simulink model "six_rod_tensegrity_model_2021a"  (R2021a)
settings: Solver=ode45  StartTime=0  StopTime=Inf  RelTol=1e-1
values from neighbouring files (symbols this model uses):
  grivity_z = -9.80665    [code_for_6_rods_tensegrity.m]
  i = 19    [drive_params.m]
  Jsum = Jd + Jp + Jnagr    (= 9.27e-08)    [drive_params.m]
  km = 9.32 / 1000    (= 0.00932)    [drive_params.m]
  kpdr = 0.81    [drive_params.m]
  kw = 60 / (2*pi * 1020)    (= 0.00936205547599)    [drive_params.m]
  L = 0.14 / 1000    (= 0.00014)    [drive_params.m]
  load_mass = 0.5    [code_for_6_rods_tensegrity.m]
  plane_offset = -(rod_length/2 + 0.032 + rod_radius)    [code_for_6_rods_tensegrity.m]
  R = 5.3    [drive_params.m]
  rod_end_drive_offset = spool_active_length    (= 0.015)    [code_for_6_rods_tensegrity.m]
  rod_end_mass = 0.05    [code_for_6_rods_tensegrity.m]
  rod_end_mass_with_drive = 0.2    [code_for_6_rods_tensegrity.m]
  rod_mass = 0.028    [code_for_6_rods_tensegrity.m]
  rod_mass_with_drive = 0.038    [code_for_6_rods_tensegrity.m]
  rod_radius = 0.004    [code_for_6_rods_tensegrity.m]
undefined symbols (not defined in the file or in its folder): Left_end_cap_1_1, Left_end_cap_2_3, Left_end_cap_3_5, Left_end_cap_4_7, Left_end_cap_5_9, Left_end_cap_6_11, Right_end_cap_1_2, Right_end_cap_2_4, Right_end_cap_3_6, Right_end_cap_4_8, Right_end_cap_5_10, Right_end_cap_6_12, Rod_center_1, Rod_center_2, Rod_center_3, Rod_center_4, Rod_center_5, Rod_center_6, sigbuilder_block, X, Y, Z
libraries: sm_lib x403, nesl_utility x73
(part 3 of 5)

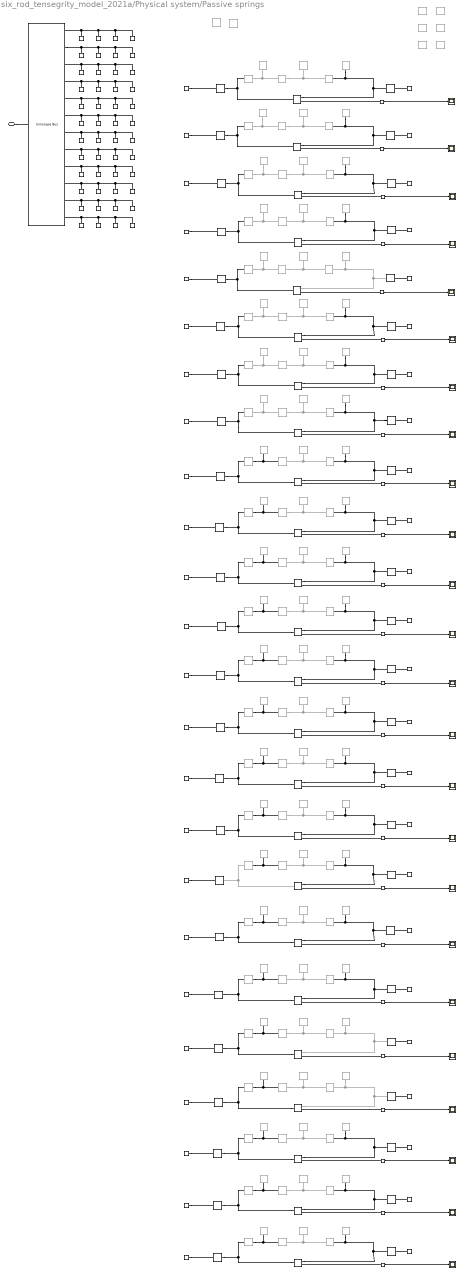
== system six_rod_tensegrity_model_2021a/Physical system/Passive springs ==
  note: Springs to passive rod
  note: Springs to active rod
  note: Springs to active rod
  note: Springs to passive rod
  note: Springs to passive rod
  note: Springs to active rod
  Cable properties {1..24} (24 alike) : sm_lib/Belts and Cables/Belt-Cable Properties  Commented=on  DrumBeltCableAlignment=Unrestricted  GraphicType=PitchLine  GraphicVisPropType=SimpleVisualProperties  GraphicDiffuseColor=cable_passive_color  GraphicSpecularColor=[0.5 0.5 0.5 1.0]  GraphicAmbientColor=[0.15 0.15 0.15 1.0]  GraphicEmissiveColor=[0.0 0.0 0.0 1.0]  GraphicShininess=75  GraphicOpacity=1
      settings: SourceProductBaseCode=MS
  Cable end {1..24} (24 alike) : sm_lib/Belts and Cables/Belt-Cable End  Commented=on
      settings: SourceProductBaseCode=MS
  Connection Label : ConnectionLabel  Label=Spring_left_1_1
  Connection Label1 : ConnectionLabel  Label=Spring_left_1_1
  Connection Label10 : ConnectionLabel  Label=Spring_left_7_2
  Connection Label11 : ConnectionLabel  Label=Spring_left_8_2
  Connection Label12 : ConnectionLabel  Label=Spring_left_7_2
  Connection Label13 : ConnectionLabel  Label=Spring_left_8_2
  Connection Label14 : ConnectionLabel  Label=Spring_left_5_2
  Connection Label15 : ConnectionLabel  Label=Spring_left_6_2
  Connection Label16 : ConnectionLabel  Label=Spring_left_9_3
  Connection Label17 : ConnectionLabel  Label=Spring_left_10_3
  Connection Label18 : ConnectionLabel  Label=Spring_left_11_3
  Connection Label19 : ConnectionLabel  Label=Spring_left_12_3
  Connection Label2 : ConnectionLabel  Label=Spring_left_2_1
  Connection Label20 : ConnectionLabel  Label=Spring_left_9_3
  Connection Label21 : ConnectionLabel  Label=Spring_left_10_3
  Connection Label22 : ConnectionLabel  Label=Spring_left_11_3
  Connection Label23 : ConnectionLabel  Label=Spring_left_12_3
  Connection Label24 : ConnectionLabel  Label=Spring_left_13_4
  Connection Label25 : ConnectionLabel  Label=Spring_left_14_4
  Connection Label26 : ConnectionLabel  Label=Spring_left_15_4
  Connection Label27 : ConnectionLabel  Label=Spring_left_16_4
  Connection Label28 : ConnectionLabel  Label=Spring_left_13_4
  Connection Label29 : ConnectionLabel  Label=Spring_left_14_4
  Connection Label3 : ConnectionLabel  Label=Spring_left_3_1
  Connection Label30 : ConnectionLabel  Label=Spring_left_15_4
  Connection Label31 : ConnectionLabel  Label=Spring_left_16_4
  Connection Label32 : ConnectionLabel  Label=Spring_left_17_5
  Connection Label33 : ConnectionLabel  Label=Spring_left_18_5
  Connection Label34 : ConnectionLabel  Label=Spring_left_19_6
  Connection Label35 : ConnectionLabel  Label=Spring_left_17_5
  Connection Label36 : ConnectionLabel  Label=Spring_left_18_5
  Connection Label37 : ConnectionLabel  Label=Spring_left_20_6
  Connection Label38 : ConnectionLabel  Label=Spring_left_19_6
  Connection Label39 : ConnectionLabel  Label=Spring_left_20_6
  Connection Label4 : ConnectionLabel  Label=Spring_left_4_1
  Connection Label40 : ConnectionLabel  Label=Spring_left_21_7
  Connection Label41 : ConnectionLabel  Label=Spring_left_22_7
  Connection Label42 : ConnectionLabel  Label=Spring_left_23_8
  Connection Label43 : ConnectionLabel  Label=Spring_left_24_8
  Connection Label44 : ConnectionLabel  Label=Spring_left_21_7
  Connection Label45 : ConnectionLabel  Label=Spring_left_22_7
  Connection Label46 : ConnectionLabel  Label=Spring_left_23_8
  Connection Label47 : ConnectionLabel  Label=Spring_left_24_8
  Connection Label48 : ConnectionLabel  Label=Spring_right_24_10
  Connection Label49 : ConnectionLabel  Label=Spring_right_23_9
  Connection Label5 : ConnectionLabel  Label=Spring_left_2_1
  Connection Label50 : ConnectionLabel  Label=Spring_right_22_12
  Connection Label51 : ConnectionLabel  Label=Spring_right_21_11
  Connection Label52 : ConnectionLabel  Label=Spring_right_20_10
  Connection Label53 : ConnectionLabel  Label=Spring_right_19_9
  Connection Label54 : ConnectionLabel  Label=Spring_right_18_12
  Connection Label55 : ConnectionLabel  Label=Spring_right_24_10
  Connection Label56 : ConnectionLabel  Label=Spring_right_23_9
  Connection Label57 : ConnectionLabel  Label=Spring_right_22_12
  Connection Label58 : ConnectionLabel  Label=Spring_right_21_11
  Connection Label59 : ConnectionLabel  Label=Spring_right_20_10
  Connection Label6 : ConnectionLabel  Label=Spring_left_3_1
  Connection Label60 : ConnectionLabel  Label=Spring_right_19_9
  Connection Label61 : ConnectionLabel  Label=Spring_right_18_12
  Connection Label62 : ConnectionLabel  Label=Spring_right_17_11
  Connection Label63 : ConnectionLabel  Label=Spring_right_16_12
  Connection Label64 : ConnectionLabel  Label=Spring_right_15_10
  Connection Label65 : ConnectionLabel  Label=Spring_right_14_8
  Connection Label66 : ConnectionLabel  Label=Spring_right_13_7
  Connection Label67 : ConnectionLabel  Label=Spring_right_12_12
  Connection Label68 : ConnectionLabel  Label=Spring_right_11_10
  Connection Label69 : ConnectionLabel  Label=Spring_right_10_6
  Connection Label7 : ConnectionLabel  Label=Spring_left_4_1
  Connection Label70 : ConnectionLabel  Label=Spring_right_9_5
  Connection Label71 : ConnectionLabel  Label=Spring_right_8_11
  Connection Label72 : ConnectionLabel  Label=Spring_right_7_9
  Connection Label73 : ConnectionLabel  Label=Spring_right_6_8
  Connection Label74 : ConnectionLabel  Label=Spring_right_5_7
  Connection Label75 : ConnectionLabel  Label=Spring_right_4_11
  Connection Label76 : ConnectionLabel  Label=Spring_right_3_9
  Connection Label77 : ConnectionLabel  Label=Spring_right_2_6
  Connection Label78 : ConnectionLabel  Label=Spring_right_1_5
  Connection Label79 : ConnectionLabel  Label=Spring_right_17_11
  Connection Label8 : ConnectionLabel  Label=Spring_left_5_2
  Connection Label80 : ConnectionLabel  Label=Spring_right_16_12
  Connection Label81 : ConnectionLabel  Label=Spring_right_15_10
  Connection Label82 : ConnectionLabel  Label=Spring_right_14_8
  Connection Label83 : ConnectionLabel  Label=Spring_right_13_7
  Connection Label84 : ConnectionLabel  Label=Spring_right_12_12
  Connection Label85 : ConnectionLabel  Label=Spring_right_11_10
  Connection Label86 : ConnectionLabel  Label=Spring_right_10_6
  Connection Label87 : ConnectionLabel  Label=Spring_right_9_5
  Connection Label88 : ConnectionLabel  Label=Spring_right_8_11
  Connection Label89 : ConnectionLabel  Label=Spring_right_7_9
  Connection Label9 : ConnectionLabel  Label=Spring_left_6_2
  Connection Label90 : ConnectionLabel  Label=Spring_right_6_8
  Connection Label91 : ConnectionLabel  Label=Spring_right_5_7
  Connection Label92 : ConnectionLabel  Label=Spring_right_4_11
  Connection Label93 : ConnectionLabel  Label=Spring_right_3_9
  Connection Label94 : ConnectionLabel  Label=Spring_right_2_6
  Connection Label95 : ConnectionLabel  Label=Spring_right_1_5
  End sphere {1..24} (24 alike) : sm_lib/Body Elements/Spherical Solid  Commented=on  GraphicAmbientColor=[0.15 0.15 0.15 1.0]  BasedOnType=Density  CenterOfMass=[0 0 0]  CenterOfMassUnits=m  GraphicDiffuseColor=spool_passive_color  Density=spool_passive_density  DensityUnits=kg/m^3  DoExposeReferenceFrame=on  GraphicEmissiveColor=[0.0 0.0 0.0 1.0]  ExportEntireGeometry=off  SerializedExposedGeometries=<ExposedGeometries/>  SerializedFrames=<Frames/>  MarkerShape=Frame  MarkerSize=10  GraphicType=FromGeometry  InertiaType=CalculateFromGeometry  Mass=0.01  MassUnits=kg  MomentsOfInertia=[1 1 1]  MomentsOfInertiaUnits=kg*m^2  GraphicOpacity=1.0  ProductsOfInertia=[0 0 0]  ProductsOfInertiaUnits=kg*m^2  GraphicShininess=10  GraphicSpecularColor=[0.8 0.8 0.8]  SphereRadius=spool_passive_radius  SphereRadiusUnits=m  GraphicVisPropType=SimpleVisualProperties
  PS-Simulink Converter{1..24} (24 alike) : nesl_utility/PS-Simulink Converter  PhysicalDomain=network_engine_domain  SubClassName=ps_output  LeftPortType=input  RightPortType=output  PseudoPeriodic=off  Frequencies=[]  Unit=N  AffineConversion=off
      settings: SourceProductBaseCode=PW,SS
  Revolute Joint {1..24} (24 alike) : sm_lib/Joints/Revolute Joint  Commented=on  JointMode=Normal  SenseConstraintForce=off  SenseConstraintForceX=off  SenseConstraintForceY=off  SenseConstraintForceZ=off  SenseConstraintTorque=off  SenseConstraintTorqueX=off  SenseConstraintTorqueY=off  SenseConstraintTorqueZ=off  SenseTotalForce=off  SenseTotalForceX=off  SenseTotalForceY=off  SenseTotalForceZ=off  SenseTotalTorque=off  SenseTotalTorqueX=off  SenseTotalTorqueY=off  SenseTotalTorqueZ=off  CompositeWrenchDir=FollowerOnBase  CompositeWrenchFrame=BaseFrame  EquilibriumPosition=0  EquilibriumPositionUnits=deg  SpringStiffness=0  SpringStiffnessUnits=N*m/deg  DampingCoefficient=0  DampingCoefficientUnits=N*m/(deg/s)  TorqueActuationMode=NoTorque  MotionActuationMode=ComputedMotion  SensePosition=off  SenseVelocity=off  SenseAcceleration=off  SenseTorqueForce=off  SenseLowerLimitTorqueForce=off  SenseUpperLimitTorqueForce=off  LowerLimitSpecify=off  LowerLimitBound=-90  LowerLimitBoundUnits=deg  LowerLimitStiffness=1e4  LowerLimitStiffnessUnits=N*m/deg  LowerLimitDamping=10  LowerLimitDampingUnits=N*m/(deg/s)  LowerLimitTransitionRegionWidth=0.1  LowerLimitTransitionRegionWidthUnits=deg  UpperLimitSpecify=off  UpperLimitBound=90  UpperLimitBoundUnits=deg  UpperLimitStiffness=1e4  UpperLimitStiffnessUnits=N*m/deg  UpperLimitDamping=10  UpperLimitDampingUnits=N*m/(deg/s)  UpperLimitTransitionRegionWidth=0.1  UpperLimitTransitionRegionWidthUnits=deg  PositionTargetSpecify=off  PositionTargetPriority=High  PositionTargetValue=0  PositionTargetValueUnits=deg  VelocityTargetSpecify=off  VelocityTargetPriority=High  VelocityTargetValue=0  VelocityTargetValueUnits=deg/s
  Simscape Bus1 : SimscapeBus  HierarchyStrings=Left_end_cap_1_1;Right_end_cap_1_2;Left_end_cap_2_3;Right_end_cap_2_4;Left_end_cap_3_5;Right_end_cap_3_6;Left_end_cap_4_7;Right_end_cap_4_8;Left_end_cap_5_9;Right_end_cap_5_10;Left_end_cap_6_11;Right_end_cap_6_12
  Sphere 1 : sm_lib/Body Elements/Spherical Solid  Commented=on  GraphicAmbientColor=[0.15 0.15 0.15 1.0]  BasedOnType=Density  CenterOfMass=[0 0 0]  CenterOfMassUnits=m  GraphicDiffuseColor=spool_passive_color  Density=spool_passive_density  DensityUnits=kg/m^3  DoExposeReferenceFrame=on  GraphicEmissiveColor=[0.0 0.0 0.0 1.0]  ExportEntireGeometry=off  SerializedExposedGeometries=<ExposedGeometries/>  SerializedFrames=<Frames/>  MarkerShape=Frame  MarkerSize=10  GraphicType=FromGeometry  InertiaType=CalculateFromGeometry  Mass=0.01  MassUnits=kg  MomentsOfInertia=[1 1 1]  MomentsOfInertiaUnits=kg*m^2  GraphicOpacity=1.0  ProductsOfInertia=[0 0 0]  ProductsOfInertiaUnits=kg*m^2  GraphicShininess=10  GraphicSpecularColor=[0.8 0.8 0.8]  SphereRadius=spool_passive_radius  SphereRadiusUnits=m  GraphicVisPropType=SimpleVisualProperties
  Spherical Joint 1 : sm_lib/Joints/Spherical Joint  Commented=on  JointMode=Normal  SenseConstraintForce=off  SenseConstraintForceX=off  SenseConstraintForceY=off  SenseConstraintForceZ=off  SenseConstraintTorque=off  SenseConstraintTorqueX=off  SenseConstraintTorqueY=off  SenseConstraintTorqueZ=off  SenseTotalForce=off  SenseTotalForceX=off  SenseTotalForceY=off  SenseTotalForceZ=off  SenseTotalTorque=off  SenseTotalTorqueX=off  SenseTotalTorqueY=off  SenseTotalTorqueZ=off  CompositeWrenchDir=FollowerOnBase  CompositeWrenchFrame=BaseFrame  DefPosRotationMethod=None  DefPosRotationAngleUnits=deg  DefPosRotationStandardAxis=+Z  DefPosRotationAngle=0.0  DefPosRotationArbitraryAxis=[0 0 1]  DefPosFollAlignAxisA=+X  DefPosBaseAlignAxisA=+Y  DefPosFollAlignAxisB=+Y  DefPosBaseAlignAxisB=+Z  DefPosRotationSequenceAxes=FollowerAxes  DefPosRotationSequence=XYX  DefPosRotationSequenceAngles=[0 0 0]  DefPosRotationSequenceAnglesUnits=deg  DefPosRotationMatrix=[1 0 0; 0 1 0; 0 0 1]  EqPosRotationMethod=None  EqPosRotationAngleUnits=deg  EqPosRotationStandardAxis=+Z  EqPosRotationAngle=0.0  EqPosRotationArbitraryAxis=[0 0 1]  EqPosFollAlignAxisA=+X  EqPosBaseAlignAxisA=+Y  EqPosFollAlignAxisB=+Y  EqPosBaseAlignAxisB=+Z  EqPosRotationSequenceAxes=FollowerAxes  EqPosRotationSequence=XYX  EqPosRotationSequenceAngles=[0 0 0]  EqPosRotationSequenceAnglesUnits=deg  EqPosRotationMatrix=[1 0 0; 0 1 0; 0 0 1]  SpringStiffness=0  SpringStiffnessUnits=N*m/deg  DampingCoefficient=0  DampingCoefficientUnits=N*m/(deg/s)  ActuateTorqueX=off  ActuateTorqueY=off  ActuateTorqueZ=off  ActuateTorque=off  TorqueActuationMode=NoTorque  MotionActuationMode=ComputedMotion  ActuationFrame=BaseFrame  SensePosition=off  SenseVelocityX=off  SenseVelocityY=off  SenseVelocityZ=off  SenseVelocity=off  SenseAccelerationX=off  SenseAccelerationY=off  SenseAccelerationZ=off  SenseAcceleration=off  SenseTorqueX=off  SenseTorqueY=off  SenseTorqueZ=off  SenseTorqueForce=off  SenseLowerLimitTorqueMag=off  SenseUpperLimitTorqueMag=off  SensingFrame=BaseFrame  LowerLimitSpecify=off  LowerLimitBound=15  LowerLimitBoundUnits=deg  LowerLimitStiffness=1e4  LowerLimitStiffnessUnits=N*m/deg  LowerLimitDamping=10  LowerLimitDampingUnits=N*m/(deg/s)  LowerLimitTransitionRegionWidth=0.1  LowerLimitTransitionRegionWidthUnits=deg  UpperLimitSpecify=off  UpperLimitBound=45  UpperLimitBoundUnits=deg  UpperLimitStiffness=1e4  UpperLimitStiffnessUnits=N*m/deg  UpperLimitDamping=10  UpperLimitDampingUnits=N*m/(deg/s)  UpperLimitTransitionRegionWidth=0.1  UpperLimitTransitionRegionWidthUnits=deg  PositionTargetRotationMethod=None  PositionTargetRotationAngleUnits=deg  PositionTargetRotationStandardAxis=+Z  PositionTargetRotationAngle=0.0  PositionTargetRotationArbitraryAxis=[0 0 1]  PositionTargetFollAlignAxisA=+X  PositionTargetBaseAlignAxisA=+Y  PositionTargetFollAlignAxisB=+Y  PositionTargetBaseAlignAxisB=+Z  PositionTargetRotationSequenceAxes=FollowerAxes  PositionTargetRotationSequence=XYX  PositionTargetRotationSequenceAngles=[0 0 0]  PositionTargetRotationSequenceAnglesUnits=deg  PositionTargetRotationMatrix=[1 0 0; 0 1 0; 0 0 1]  PositionTargetSpecify=off  PositionTargetPriority=High  VelocityTargetValue=[0 0 0]  VelocityTargetValueUnits=deg/s  VelocityTargetSpecify=off  VelocityTargetPriority=High  VelocityTargetInFollowerFrame=on
  Spool {1..24} (24 alike) : sm_lib/Belts and Cables/Belt-Cable Spool  Commented=on  PitchRadius=spool_passive_radius  PitchRadiusUnits=m  SenseSpoolAngleA=off  SenseFleetAngleA=off
      settings: SourceProductBaseCode=MS
  Spring 1 : sm_lib/Forces and Torques/Spring and Damper Force  NaturalLength=spring_natural_length_1  NaturalLengthUnits=m  SpringStiffness=spring_stiffness  SpringStiffnessUnits=N/m  DampingCoefficient=spring_damping  DampingCoefficientUnits=N/(m/s)  SenseForce=on
  Spring 10 : sm_lib/Forces and Torques/Spring and Damper Force  NaturalLength=spring_natural_length_10  NaturalLengthUnits=m  SpringStiffness=spring_stiffness  SpringStiffnessUnits=N/m  DampingCoefficient=spring_damping  DampingCoefficientUnits=N/(m/s)  SenseForce=on
  Spring 11 : sm_lib/Forces and Torques/Spring and Damper Force  NaturalLength=spring_natural_length_11  NaturalLengthUnits=m  SpringStiffness=spring_stiffness  SpringStiffnessUnits=N/m  DampingCoefficient=spring_damping  DampingCoefficientUnits=N/(m/s)  SenseForce=on
  Spring 12 : sm_lib/Forces and Torques/Spring and Damper Force  NaturalLength=spring_natural_length_12  NaturalLengthUnits=m  SpringStiffness=spring_stiffness  SpringStiffnessUnits=N/m  DampingCoefficient=spring_damping  DampingCoefficientUnits=N/(m/s)  SenseForce=on
  Spring 13 : sm_lib/Forces and Torques/Spring and Damper Force  NaturalLength=spring_natural_length_13  NaturalLengthUnits=m  SpringStiffness=spring_stiffness  SpringStiffnessUnits=N/m  DampingCoefficient=spring_damping  DampingCoefficientUnits=N/(m/s)  SenseForce=on
  Spring 14 : sm_lib/Forces and Torques/Spring and Damper Force  NaturalLength=spring_natural_length_14  NaturalLengthUnits=m  SpringStiffness=spring_stiffness  SpringStiffnessUnits=N/m  DampingCoefficient=spring_damping  DampingCoefficientUnits=N/(m/s)  SenseForce=on
  Spring 15 : sm_lib/Forces and Torques/Spring and Damper Force  NaturalLength=spring_natural_length_15  NaturalLengthUnits=m  SpringStiffness=spring_stiffness  SpringStiffnessUnits=N/m  DampingCoefficient=spring_damping  DampingCoefficientUnits=N/(m/s)  SenseForce=on
  Spring 16 : sm_lib/Forces and Torques/Spring and Damper Force  NaturalLength=spring_natural_length_16  NaturalLengthUnits=m  SpringStiffness=spring_stiffness  SpringStiffnessUnits=N/m  DampingCoefficient=spring_damping  DampingCoefficientUnits=N/(m/s)  SenseForce=on
  Spring 17 : sm_lib/Forces and Torques/Spring and Damper Force  NaturalLength=spring_natural_length_17  NaturalLengthUnits=m  SpringStiffness=spring_stiffness  SpringStiffnessUnits=N/m  DampingCoefficient=spring_damping  DampingCoefficientUnits=N/(m/s)  SenseForce=on
  Spring 18 : sm_lib/Forces and Torques/Spring and Damper Force  NaturalLength=spring_natural_length_18  NaturalLengthUnits=m  SpringStiffness=spring_stiffness  SpringStiffnessUnits=N/m  DampingCoefficient=spring_damping  DampingCoefficientUnits=N/(m/s)  SenseForce=on
  Spring 19 : sm_lib/Forces and Torques/Spring and Damper Force  NaturalLength=spring_natural_length_19  NaturalLengthUnits=m  SpringStiffness=spring_stiffness  SpringStiffnessUnits=N/m  DampingCoefficient=spring_damping  DampingCoefficientUnits=N/(m/s)  SenseForce=on
  Spring 2 : sm_lib/Forces and Torques/Spring and Damper Force  NaturalLength=spring_natural_length_2  NaturalLengthUnits=m  SpringStiffness=spring_stiffness  SpringStiffnessUnits=N/m  DampingCoefficient=spring_damping  DampingCoefficientUnits=N/(m/s)  SenseForce=on
  Spring 20 : sm_lib/Forces and Torques/Spring and Damper Force  NaturalLength=spring_natural_length_20  NaturalLengthUnits=m  SpringStiffness=spring_stiffness  SpringStiffnessUnits=N/m  DampingCoefficient=spring_damping  DampingCoefficientUnits=N/(m/s)  SenseForce=on
  Spring 21 : sm_lib/Forces and Torques/Spring and Damper Force  NaturalLength=spring_natural_length_21  NaturalLengthUnits=m  SpringStiffness=spring_stiffness  SpringStiffnessUnits=N/m  DampingCoefficient=spring_damping  DampingCoefficientUnits=N/(m/s)  SenseForce=on
  Spring 22 : sm_lib/Forces and Torques/Spring and Damper Force  NaturalLength=spring_natural_length_22  NaturalLengthUnits=m  SpringStiffness=spring_stiffness  SpringStiffnessUnits=N/m  DampingCoefficient=spring_damping  DampingCoefficientUnits=N/(m/s)  SenseForce=on
  Spring 23 : sm_lib/Forces and Torques/Spring and Damper Force  NaturalLength=spring_natural_length_23  NaturalLengthUnits=m  SpringStiffness=spring_stiffness  SpringStiffnessUnits=N/m  DampingCoefficient=spring_damping  DampingCoefficientUnits=N/(m/s)  SenseForce=on
  Spring 24 : sm_lib/Forces and Torques/Spring and Damper Force  NaturalLength=spring_natural_length_24  NaturalLengthUnits=m  SpringStiffness=spring_stiffness  SpringStiffnessUnits=N/m  DampingCoefficient=spring_damping  DampingCoefficientUnits=N/(m/s)  SenseForce=on
  Spring 3 : sm_lib/Forces and Torques/Spring and Damper Force  NaturalLength=spring_natural_length_3  NaturalLengthUnits=m  SpringStiffness=spring_stiffness  SpringStiffnessUnits=N/m  DampingCoefficient=spring_damping  DampingCoefficientUnits=N/(m/s)  SenseForce=on
  Spring 4 : sm_lib/Forces and Torques/Spring and Damper Force  NaturalLength=spring_natural_length_4  NaturalLengthUnits=m  SpringStiffness=spring_stiffness  SpringStiffnessUnits=N/m  DampingCoefficient=spring_damping  DampingCoefficientUnits=N/(m/s)  SenseForce=on
  Spring 5 : sm_lib/Forces and Torques/Spring and Damper Force  NaturalLength=spring_natural_length_5  NaturalLengthUnits=m  SpringStiffness=spring_stiffness  SpringStiffnessUnits=N/m  DampingCoefficient=spring_damping  DampingCoefficientUnits=N/(m/s)  SenseForce=on
  Spring 6 : sm_lib/Forces and Torques/Spring and Damper Force  NaturalLength=spring_natural_length_6  NaturalLengthUnits=m  SpringStiffness=spring_stiffness  SpringStiffnessUnits=N/m  DampingCoefficient=spring_damping  DampingCoefficientUnits=N/(m/s)  SenseForce=on
  Spring 7 : sm_lib/Forces and Torques/Spring and Damper Force  NaturalLength=spring_natural_length_7  NaturalLengthUnits=m  SpringStiffness=spring_stiffness  SpringStiffnessUnits=N/m  DampingCoefficient=spring_damping  DampingCoefficientUnits=N/(m/s)  SenseForce=on
  Spring 8 : sm_lib/Forces and Torques/Spring and Damper Force  NaturalLength=spring_natural_length_8  NaturalLengthUnits=m  SpringStiffness=spring_stiffness  SpringStiffnessUnits=N/m  DampingCoefficient=spring_damping  DampingCoefficientUnits=N/(m/s)  SenseForce=on
  Spring 9 : sm_lib/Forces and Torques/Spring and Damper Force  NaturalLength=spring_natural_length_9  NaturalLengthUnits=m  SpringStiffness=spring_stiffness  SpringStiffnessUnits=N/m  DampingCoefficient=spring_damping  DampingCoefficientUnits=N/(m/s)  SenseForce=on
  Winch {1..24} (24 alike) : sm_lib/Body Elements/Cylindrical Solid  Commented=on  GraphicAmbientColor=[0.15 0.15 0.15 1.0]  BasedOnType=Density  CenterOfMass=[0 0 0]  CenterOfMassUnits=m  GraphicDiffuseColor=spool_passive_color  CylinderLength=spool_passive_length  CylinderLengthUnits=m  CylinderRadius=spool_passive_radius  CylinderRadiusUnits=m  Density=spool_passive_density  DensityUnits=kg/m^3  DoExposeReferenceFrame=on  GraphicEmissiveColor=[0.0 0.0 0.0 1.0]  ExportEntireGeometry=off  SerializedFrames=<Frames/>  MarkerShape=Frame  MarkerSize=10  GraphicType=FromGeometry  InertiaType=CalculateFromGeometry  Mass=0.01  MassUnits=kg  MomentsOfInertia=[1 1 1]  MomentsOfInertiaUnits=kg*m^2  GraphicOpacity=1.0  ProductsOfInertia=[0 0 0]  ProductsOfInertiaUnits=kg*m^2  GraphicShininess=10  GraphicSpecularColor=[0.8 0.8 0.8]  GraphicVisPropType=SimpleVisualProperties
  X+1 : sm_lib/Frames and Transforms/Rigid Transform  TranslationMethod=StandardAxis  TranslationStandardOffset=rod_radius  TranslationLengthUnit=m  TranslationStandardAxis=+X  TranslationCartesianOffset=[0 0 0]  TranslationROffset=0  TranslationROffsetUnits=m  TranslationZOffset=0  TranslationZOffsetUnits=m  TranslationThetaOffset=0  TranslationThetaOffsetUnits=deg  RotationMethod=StandardAxis  RotationAngleUnits=deg  RotationStandardAxis=-X  RotationAngle=90  RotationArbitraryAxis=[0 0 1]  FollAlignAxisA=+X  BaseAlignAxisA=+Y  FollAlignAxisB=+Y  BaseAlignAxisB=+Z  RotationSequenceAxes=FollowerAxes  RotationSequence=XYX  RotationSequenceAngles=[0 0 0]  RotationSequenceAnglesUnits=deg  RotationMatrix=[1 0 0; 0 1 0; 0 0 1]
  X+{4..12} (9 alike) : sm_lib/Frames and Transforms/Rigid Transform  TranslationMethod=StandardAxis  TranslationStandardOffset=rod_radius  TranslationLengthUnit=m  TranslationStandardAxis=+X  TranslationCartesianOffset=[0 0 0]  TranslationROffset=0  TranslationROffsetUnits=m  TranslationZOffset=0  TranslationZOffsetUnits=m  TranslationThetaOffset=0  TranslationThetaOffsetUnits=deg  RotationMethod=None  RotationAngleUnits=deg  RotationStandardAxis=+Z  RotationAngle=0.0  RotationArbitraryAxis=[0 0 1]  FollAlignAxisA=+X  BaseAlignAxisA=+Y  FollAlignAxisB=+Y  BaseAlignAxisB=+Z  RotationSequenceAxes=FollowerAxes  RotationSequence=XYX  RotationSequenceAngles=[0 0 0]  RotationSequenceAnglesUnits=deg  RotationMatrix=[1 0 0; 0 1 0; 0 0 1]
  X+2 : sm_lib/Frames and Transforms/Rigid Transform  TranslationMethod=StandardAxis  TranslationStandardOffset=rod_radius  TranslationLengthUnit=m  TranslationStandardAxis=+X  TranslationCartesianOffset=[0 0 0]  TranslationROffset=0  TranslationROffsetUnits=m  TranslationZOffset=0  TranslationZOffsetUnits=m  TranslationThetaOffset=0  TranslationThetaOffsetUnits=deg  RotationMethod=StandardAxis  RotationAngleUnits=deg  RotationStandardAxis=+X  RotationAngle=90  RotationArbitraryAxis=[0 0 1]  FollAlignAxisA=+X  BaseAlignAxisA=+Y  FollAlignAxisB=+Y  BaseAlignAxisB=+Z  RotationSequenceAxes=FollowerAxes  RotationSequence=XYX  RotationSequenceAngles=[0 0 0]  RotationSequenceAnglesUnits=deg  RotationMatrix=[1 0 0; 0 1 0; 0 0 1]
  X+3 : sm_lib/Frames and Transforms/Rigid Transform  TranslationMethod=StandardAxis  TranslationStandardOffset=rod_radius  TranslationLengthUnit=m  TranslationStandardAxis=+X  TranslationCartesianOffset=[0 0 0]  TranslationROffset=0  TranslationROffsetUnits=m  TranslationZOffset=0  TranslationZOffsetUnits=m  TranslationThetaOffset=0  TranslationThetaOffsetUnits=deg  RotationMethod=StandardAxis  RotationAngleUnits=deg  RotationStandardAxis=-X  RotationAngle=90  RotationArbitraryAxis=[0 0 1]  FollAlignAxisA=+X  BaseAlignAxisA=+Y  FollAlignAxisB=+Y  BaseAlignAxisB=+Z  RotationSequenceAxes=FollowerAxes  RotationSequence=XYX  RotationSequenceAngles=[0 0 0]  RotationSequenceAnglesUnits=deg  RotationMatrix=[1 0 0; 0 1 0; 0 0 1]
  X+Temp : sm_lib/Frames and Transforms/Rigid Transform  Commented=on  TranslationMethod=StandardAxis  TranslationStandardOffset=rod_radius  TranslationLengthUnit=m  TranslationStandardAxis=+X  TranslationCartesianOffset=[0 0 0]  TranslationROffset=0  TranslationROffsetUnits=m  TranslationZOffset=0  TranslationZOffsetUnits=m  TranslationThetaOffset=0  TranslationThetaOffsetUnits=deg  RotationMethod=None  RotationAngleUnits=deg  RotationStandardAxis=+Z  RotationAngle=0.0  RotationArbitraryAxis=[0 0 1]  FollAlignAxisA=+X  BaseAlignAxisA=+Y  FollAlignAxisB=+Y  BaseAlignAxisB=+Z  RotationSequenceAxes=FollowerAxes  RotationSequence=XYX  RotationSequenceAngles=[0 0 0]  RotationSequenceAnglesUnits=deg  RotationMatrix=[1 0 0; 0 1 0; 0 0 1]
  X-1 : sm_lib/Frames and Transforms/Rigid Transform  TranslationMethod=StandardAxis  TranslationStandardOffset=rod_radius  TranslationLengthUnit=m  TranslationStandardAxis=-X  TranslationCartesianOffset=[0 0 0]  TranslationROffset=0  TranslationROffsetUnits=m  TranslationZOffset=0  TranslationZOffsetUnits=m  TranslationThetaOffset=0  TranslationThetaOffsetUnits=deg  RotationMethod=StandardAxis  RotationAngleUnits=deg  RotationStandardAxis=+X  RotationAngle=90  RotationArbitraryAxis=[0 0 1]  FollAlignAxisA=+X  BaseAlignAxisA=+Y  FollAlignAxisB=+Y  BaseAlignAxisB=+Z  RotationSequenceAxes=FollowerAxes  RotationSequence=XYX  RotationSequenceAngles=[0 0 0]  RotationSequenceAnglesUnits=deg  RotationMatrix=[1 0 0; 0 1 0; 0 0 1]
  X-{4..12} (9 alike) : sm_lib/Frames and Transforms/Rigid Transform  TranslationMethod=StandardAxis  TranslationStandardOffset=rod_radius  TranslationLengthUnit=m  TranslationStandardAxis=-X  TranslationCartesianOffset=[0 0 0]  TranslationROffset=0  TranslationROffsetUnits=m  TranslationZOffset=0  TranslationZOffsetUnits=m  TranslationThetaOffset=0  TranslationThetaOffsetUnits=deg  RotationMethod=None  RotationAngleUnits=deg  RotationStandardAxis=+Z  RotationAngle=0.0  RotationArbitraryAxis=[0 0 1]  FollAlignAxisA=+X  BaseAlignAxisA=+Y  FollAlignAxisB=+Y  BaseAlignAxisB=+Z  RotationSequenceAxes=FollowerAxes  RotationSequence=XYX  RotationSequenceAngles=[0 0 0]  RotationSequenceAnglesUnits=deg  RotationMatrix=[1 0 0; 0 1 0; 0 0 1]
  X-2 : sm_lib/Frames and Transforms/Rigid Transform  TranslationMethod=StandardAxis  TranslationStandardOffset=rod_radius  TranslationLengthUnit=m  TranslationStandardAxis=-X  TranslationCartesianOffset=[0 0 0]  TranslationROffset=0  TranslationROffsetUnits=m  TranslationZOffset=0  TranslationZOffsetUnits=m  TranslationThetaOffset=0  TranslationThetaOffsetUnits=deg  RotationMethod=StandardAxis  RotationAngleUnits=deg  RotationStandardAxis=-X  RotationAngle=90  RotationArbitraryAxis=[0 0 1]  FollAlignAxisA=+X  BaseAlignAxisA=+Y  FollAlignAxisB=+Y  BaseAlignAxisB=+Z  RotationSequenceAxes=FollowerAxes  RotationSequence=XYX  RotationSequenceAngles=[0 0 0]  RotationSequenceAnglesUnits=deg  RotationMatrix=[1 0 0; 0 1 0; 0 0 1]
  X-3 : sm_lib/Frames and Transforms/Rigid Transform  TranslationMethod=StandardAxis  TranslationStandardOffset=rod_radius  TranslationLengthUnit=m  TranslationStandardAxis=-X  TranslationCartesianOffset=[0 0 0]  TranslationROffset=0  TranslationROffsetUnits=m  TranslationZOffset=0  TranslationZOffsetUnits=m  TranslationThetaOffset=0  TranslationThetaOffsetUnits=deg  RotationMethod=StandardAxis  RotationAngleUnits=deg  RotationStandardAxis=+X  RotationAngle=90  RotationArbitraryAxis=[0 0 1]  FollAlignAxisA=+X  BaseAlignAxisA=+Y  FollAlignAxisB=+Y  BaseAlignAxisB=+Z  RotationSequenceAxes=FollowerAxes  RotationSequence=XYX  RotationSequenceAngles=[0 0 0]  RotationSequenceAnglesUnits=deg  RotationMatrix=[1 0 0; 0 1 0; 0 0 1]
  X-Temp : sm_lib/Frames and Transforms/Rigid Transform  Commented=on  TranslationMethod=StandardAxis  TranslationStandardOffset=rod_radius  TranslationLengthUnit=m  TranslationStandardAxis=-X  TranslationCartesianOffset=[0 0 0]  TranslationROffset=0  TranslationROffsetUnits=m  TranslationZOffset=0  TranslationZOffsetUnits=m  TranslationThetaOffset=0  TranslationThetaOffsetUnits=deg  RotationMethod=None  RotationAngleUnits=deg  RotationStandardAxis=+Z  RotationAngle=0.0  RotationArbitraryAxis=[0 0 1]  FollAlignAxisA=+X  BaseAlignAxisA=+Y  FollAlignAxisB=+Y  BaseAlignAxisB=+Z  RotationSequenceAxes=FollowerAxes  RotationSequence=XYX  RotationSequenceAngles=[0 0 0]  RotationSequenceAnglesUnits=deg  RotationMatrix=[1 0 0; 0 1 0; 0 0 1]
  Y+1 : sm_lib/Frames and Transforms/Rigid Transform  TranslationMethod=StandardAxis  TranslationStandardOffset=rod_radius  TranslationLengthUnit=m  TranslationStandardAxis=+Y  TranslationCartesianOffset=[0 0 0]  TranslationROffset=0  TranslationROffsetUnits=m  TranslationZOffset=0  TranslationZOffsetUnits=m  TranslationThetaOffset=0  TranslationThetaOffsetUnits=deg  RotationMethod=StandardAxis  RotationAngleUnits=deg  RotationStandardAxis=-Y  RotationAngle=90  RotationArbitraryAxis=[0 0 1]  FollAlignAxisA=+X  BaseAlignAxisA=+Y  FollAlignAxisB=+Y  BaseAlignAxisB=+Z  RotationSequenceAxes=FollowerAxes  RotationSequence=XYX  RotationSequenceAngles=[0 0 0]  RotationSequenceAnglesUnits=deg  RotationMatrix=[1 0 0; 0 1 0; 0 0 1]
  Y+{4,6..12} (8 alike) : sm_lib/Frames and Transforms/Rigid Transform  TranslationMethod=StandardAxis  TranslationStandardOffset=rod_radius  TranslationLengthUnit=m  TranslationStandardAxis=+Y  TranslationCartesianOffset=[0 0 0]  TranslationROffset=0  TranslationROffsetUnits=m  TranslationZOffset=0  TranslationZOffsetUnits=m  TranslationThetaOffset=0  TranslationThetaOffsetUnits=deg  RotationMethod=None  RotationAngleUnits=deg  RotationStandardAxis=+Z  RotationAngle=0.0  RotationArbitraryAxis=[0 0 1]  FollAlignAxisA=+X  BaseAlignAxisA=+Y  FollAlignAxisB=+Y  BaseAlignAxisB=+Z  RotationSequenceAxes=FollowerAxes  RotationSequence=XYX  RotationSequenceAngles=[0 0 0]  RotationSequenceAnglesUnits=deg  RotationMatrix=[1 0 0; 0 1 0; 0 0 1]
  Y+2 : sm_lib/Frames and Transforms/Rigid Transform  TranslationMethod=StandardAxis  TranslationStandardOffset=rod_radius  TranslationLengthUnit=m  TranslationStandardAxis=+Y  TranslationCartesianOffset=[0 0 0]  TranslationROffset=0  TranslationROffsetUnits=m  TranslationZOffset=0  TranslationZOffsetUnits=m  TranslationThetaOffset=0  TranslationThetaOffsetUnits=deg  RotationMethod=StandardAxis  RotationAngleUnits=deg  RotationStandardAxis=+Y  RotationAngle=90  RotationArbitraryAxis=[0 0 1]  FollAlignAxisA=+X  BaseAlignAxisA=+Y  FollAlignAxisB=+Y  BaseAlignAxisB=+Z  RotationSequenceAxes=FollowerAxes  RotationSequence=XYX  RotationSequenceAngles=[0 0 0]  RotationSequenceAnglesUnits=deg  RotationMatrix=[1 0 0; 0 1 0; 0 0 1]
  Y+3 : sm_lib/Frames and Transforms/Rigid Transform  TranslationMethod=StandardAxis  TranslationStandardOffset=rod_radius  TranslationLengthUnit=m  TranslationStandardAxis=+Y  TranslationCartesianOffset=[0 0 0]  TranslationROffset=0  TranslationROffsetUnits=m  TranslationZOffset=0  TranslationZOffsetUnits=m  TranslationThetaOffset=0  TranslationThetaOffsetUnits=deg  RotationMethod=StandardAxis  RotationAngleUnits=deg  RotationStandardAxis=-Y  RotationAngle=90  RotationArbitraryAxis=[0 0 1]  FollAlignAxisA=+X  BaseAlignAxisA=+Y  FollAlignAxisB=+Y  BaseAlignAxisB=+Z  RotationSequenceAxes=FollowerAxes  RotationSequence=XYX  RotationSequenceAngles=[0 0 0]  RotationSequenceAnglesUnits=deg  RotationMatrix=[1 0 0; 0 1 0; 0 0 1]
  Y+5 : sm_lib/Frames and Transforms/Rigid Transform  TranslationMethod=StandardAxis  TranslationStandardOffset=rod_radius  TranslationLengthUnit=m  TranslationStandardAxis=+Y  TranslationCartesianOffset=[0 0 0]  TranslationROffset=0  TranslationROffsetUnits=m  TranslationZOffset=0  TranslationZOffsetUnits=m  TranslationThetaOffset=0  TranslationThetaOffsetUnits=deg  RotationMethod=StandardAxis  RotationAngleUnits=deg  RotationStandardAxis=-Y  RotationAngle=90  RotationArbitraryAxis=[0 0 1]  FollAlignAxisA=+X  BaseAlignAxisA=+Y  FollAlignAxisB=+Y  BaseAlignAxisB=+Z  RotationSequenceAxes=FollowerAxes  RotationSequence=XYX  RotationSequenceAngles=[0 0 0]  RotationSequenceAnglesUnits=deg  RotationMatrix=[1 0 0; 0 1 0; 0 0 1]
  Y+Temp : sm_lib/Frames and Transforms/Rigid Transform  Commented=on  TranslationMethod=StandardAxis  TranslationStandardOffset=rod_radius  TranslationLengthUnit=m  TranslationStandardAxis=+Y  TranslationCartesianOffset=[0 0 0]  TranslationROffset=0  TranslationROffsetUnits=m  TranslationZOffset=0  TranslationZOffsetUnits=m  TranslationThetaOffset=0  TranslationThetaOffsetUnits=deg  RotationMethod=None  RotationAngleUnits=deg  RotationStandardAxis=+Z  RotationAngle=0.0  RotationArbitraryAxis=[0 0 1]  FollAlignAxisA=+X  BaseAlignAxisA=+Y  FollAlignAxisB=+Y  BaseAlignAxisB=+Z  RotationSequenceAxes=FollowerAxes  RotationSequence=XYX  RotationSequenceAngles=[0 0 0]  RotationSequenceAnglesUnits=deg  RotationMatrix=[1 0 0; 0 1 0; 0 0 1]
  Y-1 : sm_lib/Frames and Transforms/Rigid Transform  TranslationMethod=StandardAxis  TranslationStandardOffset=rod_radius  TranslationLengthUnit=m  TranslationStandardAxis=-Y  TranslationCartesianOffset=[0 0 0]  TranslationROffset=0  TranslationROffsetUnits=m  TranslationZOffset=0  TranslationZOffsetUnits=m  TranslationThetaOffset=0  TranslationThetaOffsetUnits=deg  RotationMethod=StandardAxis  RotationAngleUnits=deg  RotationStandardAxis=+Y  RotationAngle=90  RotationArbitraryAxis=[0 0 1]  FollAlignAxisA=+X  BaseAlignAxisA=+Y  FollAlignAxisB=+Y  BaseAlignAxisB=+Z  RotationSequenceAxes=FollowerAxes  RotationSequence=XYX  RotationSequenceAngles=[0 0 0]  RotationSequenceAnglesUnits=deg  RotationMatrix=[1 0 0; 0 1 0; 0 0 1]
  Y-{4,6..12} (8 alike) : sm_lib/Frames and Transforms/Rigid Transform  TranslationMethod=StandardAxis  TranslationStandardOffset=rod_radius  TranslationLengthUnit=m  TranslationStandardAxis=-Y  TranslationCartesianOffset=[0 0 0]  TranslationROffset=0  TranslationROffsetUnits=m  TranslationZOffset=0  TranslationZOffsetUnits=m  TranslationThetaOffset=0  TranslationThetaOffsetUnits=deg  RotationMethod=None  RotationAngleUnits=deg  RotationStandardAxis=+Z  RotationAngle=0.0  RotationArbitraryAxis=[0 0 1]  FollAlignAxisA=+X  BaseAlignAxisA=+Y  FollAlignAxisB=+Y  BaseAlignAxisB=+Z  RotationSequenceAxes=FollowerAxes  RotationSequence=XYX  RotationSequenceAngles=[0 0 0]  RotationSequenceAnglesUnits=deg  RotationMatrix=[1 0 0; 0 1 0; 0 0 1]
  Y-2 : sm_lib/Frames and Transforms/Rigid Transform  TranslationMethod=StandardAxis  TranslationStandardOffset=rod_radius  TranslationLengthUnit=m  TranslationStandardAxis=-Y  TranslationCartesianOffset=[0 0 0]  TranslationROffset=0  TranslationROffsetUnits=m  TranslationZOffset=0  TranslationZOffsetUnits=m  TranslationThetaOffset=0  TranslationThetaOffsetUnits=deg  RotationMethod=StandardAxis  RotationAngleUnits=deg  RotationStandardAxis=-Y  RotationAngle=90  RotationArbitraryAxis=[0 0 1]  FollAlignAxisA=+X  BaseAlignAxisA=+Y  FollAlignAxisB=+Y  BaseAlignAxisB=+Z  RotationSequenceAxes=FollowerAxes  RotationSequence=XYX  RotationSequenceAngles=[0 0 0]  RotationSequenceAnglesUnits=deg  RotationMatrix=[1 0 0; 0 1 0; 0 0 1]
  Y-3 : sm_lib/Frames and Transforms/Rigid Transform  TranslationMethod=StandardAxis  TranslationStandardOffset=rod_radius  TranslationLengthUnit=m  TranslationStandardAxis=-Y  TranslationCartesianOffset=[0 0 0]  TranslationROffset=0  TranslationROffsetUnits=m  TranslationZOffset=0  TranslationZOffsetUnits=m  TranslationThetaOffset=0  TranslationThetaOffsetUnits=deg  RotationMethod=StandardAxis  RotationAngleUnits=deg  RotationStandardAxis=+Y  RotationAngle=90  RotationArbitraryAxis=[0 0 1]  FollAlignAxisA=+X  BaseAlignAxisA=+Y  FollAlignAxisB=+Y  BaseAlignAxisB=+Z  RotationSequenceAxes=FollowerAxes  RotationSequence=XYX  RotationSequenceAngles=[0 0 0]  RotationSequenceAnglesUnits=deg  RotationMatrix=[1 0 0; 0 1 0; 0 0 1]
  Y-5 : sm_lib/Frames and Transforms/Rigid Transform  TranslationMethod=StandardAxis  TranslationStandardOffset=rod_radius  TranslationLengthUnit=m  TranslationStandardAxis=-Y  TranslationCartesianOffset=[0 0 0]  TranslationROffset=0  TranslationROffsetUnits=m  TranslationZOffset=0  TranslationZOffsetUnits=m  TranslationThetaOffset=0  TranslationThetaOffsetUnits=deg  RotationMethod=StandardAxis  RotationAngleUnits=deg  RotationStandardAxis=-Y  RotationAngle=90  RotationArbitraryAxis=[0 0 1]  FollAlignAxisA=+X  BaseAlignAxisA=+Y  FollAlignAxisB=+Y  BaseAlignAxisB=+Z  RotationSequenceAxes=FollowerAxes  RotationSequence=XYX  RotationSequenceAngles=[0 0 0]  RotationSequenceAnglesUnits=deg  RotationMatrix=[1 0 0; 0 1 0; 0 0 1]
  Y-Temp : sm_lib/Frames and Transforms/Rigid Transform  Commented=on  TranslationMethod=StandardAxis  TranslationStandardOffset=rod_radius  TranslationLengthUnit=m  TranslationStandardAxis=-Y  TranslationCartesianOffset=[0 0 0]  TranslationROffset=0  TranslationROffsetUnits=m  TranslationZOffset=0  TranslationZOffsetUnits=m  TranslationThetaOffset=0  TranslationThetaOffsetUnits=deg  RotationMethod=None  RotationAngleUnits=deg  RotationStandardAxis=+Z  RotationAngle=0.0  RotationArbitraryAxis=[0 0 1]  FollAlignAxisA=+X  BaseAlignAxisA=+Y  FollAlignAxisB=+Y  BaseAlignAxisB=+Z  RotationSequenceAxes=FollowerAxes  RotationSequence=XYX  RotationSequenceAngles=[0 0 0]  RotationSequenceAnglesUnits=deg  RotationMatrix=[1 0 0; 0 1 0; 0 0 1]
  Z+Temp : sm_lib/Frames and Transforms/Rigid Transform  Commented=on  TranslationMethod=StandardAxis  TranslationStandardOffset=rod_radius  TranslationLengthUnit=m  TranslationStandardAxis=+Z  TranslationCartesianOffset=[0 0 0]  TranslationROffset=0  TranslationROffsetUnits=m  TranslationZOffset=0  TranslationZOffsetUnits=m  TranslationThetaOffset=0  TranslationThetaOffsetUnits=deg  RotationMethod=None  RotationAngleUnits=deg  RotationStandardAxis=+Z  RotationAngle=0.0  RotationArbitraryAxis=[0 0 1]  FollAlignAxisA=+X  BaseAlignAxisA=+Y  FollAlignAxisB=+Y  BaseAlignAxisB=+Z  RotationSequenceAxes=FollowerAxes  RotationSequence=XYX  RotationSequenceAngles=[0 0 0]  RotationSequenceAnglesUnits=deg  RotationMatrix=[1 0 0; 0 1 0; 0 0 1]
  Z-Temp : sm_lib/Frames and Transforms/Rigid Transform  Commented=on  TranslationMethod=StandardAxis  TranslationStandardOffset=rod_radius  TranslationLengthUnit=m  TranslationStandardAxis=-Z  TranslationCartesianOffset=[0 0 0]  TranslationROffset=0  TranslationROffsetUnits=m  TranslationZOffset=0  TranslationZOffsetUnits=m  TranslationThetaOffset=0  TranslationThetaOffsetUnits=deg  RotationMethod=None  RotationAngleUnits=deg  RotationStandardAxis=+Z  RotationAngle=0.0  RotationArbitraryAxis=[0 0 1]  FollAlignAxisA=+X  BaseAlignAxisA=+Y  FollAlignAxisB=+Y  BaseAlignAxisB=+Z  RotationSequenceAxes=FollowerAxes  RotationSequence=XYX  RotationSequenceAngles=[0 0 0]  RotationSequenceAnglesUnits=deg  RotationMatrix=[1 0 0; 0 1 0; 0 0 1]
  spring force {1..24} (24 alike) : Scope
  Rods end caps bus : PMIOPort  Side=Left
  wires:
  PS-Simulink Converter1/1 -> spring force 1/1
  PS-Simulink Converter2/1 -> spring force 2/1
  PS-Simulink Converter3/1 -> spring force 3/1
  PS-Simulink Converter4/1 -> spring force 4/1
  PS-Simulink Converter5/1 -> spring force 5/1
  PS-Simulink Converter6/1 -> spring force 6/1
  PS-Simulink Converter7/1 -> spring force 7/1
  PS-Simulink Converter8/1 -> spring force 8/1
  PS-Simulink Converter9/1 -> spring force 9/1
  PS-Simulink Converter10/1 -> spring force 10/1
  PS-Simulink Converter11/1 -> spring force 11/1
  PS-Simulink Converter12/1 -> spring force 12/1
  PS-Simulink Converter13/1 -> spring force 13/1
  PS-Simulink Converter14/1 -> spring force 14/1
  PS-Simulink Converter15/1 -> spring force 15/1
  PS-Simulink Converter16/1 -> spring force 16/1
  PS-Simulink Converter17/1 -> spring force 17/1
  PS-Simulink Converter18/1 -> spring force 18/1
  PS-Simulink Converter19/1 -> spring force 19/1
  PS-Simulink Converter20/1 -> spring force 20/1
  PS-Simulink Converter21/1 -> spring force 21/1
  PS-Simulink Converter22/1 -> spring force 22/1
  PS-Simulink Converter23/1 -> spring force 23/1
  PS-Simulink Converter24/1 -> spring force 24/1
  connections:
  Connection Label/LConn1 -- Y+1/LConn1
  Connection Label3/LConn1 -- Y-1/LConn1
  Connection Label4/LConn1 -- X-1/LConn1
  Connection Label8/LConn1 -- Y+2/LConn1
  Connection Label10/LConn1 -- Y-2/LConn1
  Connection Label11/LConn1 -- X-2/LConn1
  Connection Label2/LConn1 -- X+1/LConn1
  Connection Label9/LConn1 -- X+2/LConn1
  Y+1/RConn1 -- Revolute Joint 1/LConn1 -- Spring 1/LConn1
  Spool 1/RConn1 -- Cable end 1/RConn1 -- Cable properties 1/LConn1
  Spool 1/LConn1 -- Revolute Joint 1/RConn1 -- Winch 1/RConn1
  Spring 1/RConn1 -- Y-5/RConn1 -- End sphere 1/RConn1 -- Cable end 1/LConn1
  PS-Simulink Converter1/LConn1 -- Spring 1/RConn2
  X+1/RConn1 -- Revolute Joint 2/LConn1 -- Spring 2/LConn1
  Y-6/RConn1 -- Spring 2/RConn1 -- End sphere 2/RConn1 -- Cable end 2/LConn1
  Spool 2/RConn1 -- Cable end 2/RConn1 -- Cable properties 2/LConn1
  Spool 2/LConn1 -- Revolute Joint 2/RConn1 -- Winch 2/RConn1
  PS-Simulink Converter2/LConn1 -- Spring 2/RConn2
  Y-1/RConn1 -- Revolute Joint 3/LConn1 -- Spring 3/LConn1
  Connection Label76/LConn1 -- X+9/LConn1
  Spool 3/RConn1 -- Cable end 3/RConn1 -- Cable properties 3/LConn1
  Spool 3/LConn1 -- Winch 3/RConn1 -- Revolute Joint 3/RConn1
  PS-Simulink Converter3/LConn1 -- Spring 3/RConn2
  X-1/RConn1 -- Revolute Joint 4/LConn1 -- Spring 4/LConn1
  Spring 4/RConn1 -- End sphere 4/RConn1 -- Cable end 4/LConn1 -- X-11/RConn1
  Spool 4/RConn1 -- Cable end 4/RConn1 -- Cable properties 4/LConn1
  Spool 4/LConn1 -- Winch 4/RConn1 -- Revolute Joint 4/RConn1
  PS-Simulink Converter4/LConn1 -- Spring 4/RConn2
  Y+2/RConn1 -- Revolute Joint 5/LConn1 -- Spring 5/LConn1
  Connection Label74/LConn1 -- X-7/LConn1
  Spool 5/RConn1 -- Cable end 5/RConn1 -- Cable properties 5/LConn1
  Spool 5/LConn1 -- Winch 5/RConn1 -- Revolute Joint 5/RConn1
  PS-Simulink Converter5/LConn1 -- Spring 5/RConn2
  X+2/RConn1 -- Revolute Joint 6/LConn1 -- Spring 6/LConn1
  Connection Label73/LConn1 -- X-8/LConn1
  Spool 6/RConn1 -- Cable end 6/RConn1 -- Cable properties 6/LConn1
  Spool 6/LConn1 -- Revolute Joint 6/RConn1 -- Winch 6/RConn1
  PS-Simulink Converter6/LConn1 -- Spring 6/RConn2
  Y-2/RConn1 -- Revolute Joint 7/LConn1 -- Spring 7/LConn1
  Y+9/RConn1 -- Spring 7/RConn1 -- End sphere 7/RConn1 -- Cable end 7/LConn1
  Spool 7/RConn1 -- Cable end 7/RConn1 -- Cable properties 7/LConn1
  Spool 7/LConn1 -- Winch 7/RConn1 -- Revolute Joint 7/RConn1
  PS-Simulink Converter7/LConn1 -- Spring 7/RConn2
  X-2/RConn1 -- Revolute Joint 8/LConn1 -- Spring 8/LConn1
  Connection Label71/LConn1 -- Y+11/LConn1
  Spool 8/RConn1 -- Cable end 8/RConn1 -- Cable properties 8/LConn1
  Spool 8/LConn1 -- Winch 8/RConn1 -- Revolute Joint 8/RConn1
  PS-Simulink Converter8/LConn1 -- Spring 8/RConn2
  Spring 9/LConn1 -- Y+3/RConn1 -- Revolute Joint 9/LConn1
  Connection Label70/LConn1 -- Y+5/LConn1
  Spool 9/RConn1 -- Cable end 9/RConn1 -- Cable properties 9/LConn1
  Winch 9/RConn1 -- Revolute Joint 9/RConn1 -- Spool 9/LConn1
  PS-Simulink Converter9/LConn1 -- Spring 9/RConn2
  Spring 10/LConn1 -- X-3/RConn1 -- Revolute Joint 10/LConn1
  Spring 10/RConn1 -- X+6/RConn1 -- End sphere 10/RConn1 -- Cable end 10/LConn1
  Spool 10/RConn1 -- Cable end 10/RConn1 -- Cable properties 10/LConn1
  Winch 10/RConn1 -- Revolute Joint 10/RConn1 -- Spool 10/LConn1
  PS-Simulink Converter10/LConn1 -- Spring 10/RConn2
  Spring 11/LConn1 -- Y-3/RConn1 -- Revolute Joint 11/LConn1
  Y-10/RConn1 -- Spring 11/RConn1 -- End sphere 11/RConn1 -- Cable end 11/LConn1
  Spool 11/RConn1 -- Cable end 11/RConn1 -- Cable properties 11/LConn1
  Winch 11/RConn1 -- Revolute Joint 11/RConn1 -- Spool 11/LConn1
  PS-Simulink Converter11/LConn1 -- Spring 11/RConn2
  Spring 12/LConn1 -- X+3/RConn1 -- Revolute Joint 12/LConn1
  Y-12/RConn1 -- Spring 12/RConn1 -- End sphere 12/RConn1 -- Cable end 12/LConn1
  Spool 12/RConn1 -- Cable end 12/RConn1 -- Cable properties 12/LConn1
  Winch 12/RConn1 -- Revolute Joint 12/RConn1 -- Spool 12/LConn1
  PS-Simulink Converter12/LConn1 -- Spring 12/RConn2
  Spring 13/LConn1 -- Y+4/RConn1 -- Revolute Joint 13/LConn1
  Y+7/RConn1 -- Spring 13/RConn1 -- End sphere 13/RConn1 -- Cable end 13/LConn1
  Spool 13/RConn1 -- Cable end 13/RConn1 -- Cable properties 13/LConn1
  Winch 13/RConn1 -- Revolute Joint 13/RConn1 -- Spool 13/LConn1
  PS-Simulink Converter13/LConn1 -- Spring 13/RConn2
  Spring 14/LConn1 -- X-4/RConn1 -- Revolute Joint 14/LConn1
  Y+8/RConn1 -- Spring 14/RConn1 -- End sphere 14/RConn1 -- Cable end 14/LConn1
  Spool 14/RConn1 -- Cable end 14/RConn1 -- Cable properties 14/LConn1
  Winch 14/RConn1 -- Revolute Joint 14/RConn1 -- Spool 14/LConn1
  PS-Simulink Converter14/LConn1 -- Spring 14/RConn2
  Spring 15/LConn1 -- Y-4/RConn1 -- Revolute Joint 15/LConn1
  X+10/RConn1 -- Spring 15/RConn1 -- End sphere 15/RConn1 -- Cable end 15/LConn1
  Spool 15/RConn1 -- Cable end 15/RConn1 -- Cable properties 15/LConn1
  Winch 15/RConn1 -- Revolute Joint 15/RConn1 -- Spool 15/LConn1
  PS-Simulink Converter15/LConn1 -- Spring 15/RConn2
  Connection Label27/LConn1 -- X+4/LConn1
  X-12/RConn1 -- Spring 16/RConn1 -- End sphere 16/RConn1 -- Cable end 16/LConn1
  Spool 16/RConn1 -- Cable end 16/RConn1 -- Cable properties 16/LConn1
  Winch 16/RConn1 -- Revolute Joint 16/RConn1 -- Spool 16/LConn1
  PS-Simulink Converter16/LConn1 -- Spring 16/RConn2
  Connection Label62/LConn1 -- Y-11/LConn1
  Spool 17/RConn1 -- Cable end 17/RConn1 -- Cable properties 17/LConn1
  Winch 17/RConn1 -- Revolute Joint 17/RConn1 -- Spool 17/LConn1
  PS-Simulink Converter17/LConn1 -- Spring 17/RConn2
  Spring 18/LConn1 -- X+5/RConn1 -- Revolute Joint 18/LConn1
  Connection Label54/LConn1 -- X+12/LConn1
  Spool 18/RConn1 -- Cable end 18/RConn1 -- Cable properties 18/LConn1
  Winch 18/RConn1 -- Revolute Joint 18/RConn1 -- Spool 18/LConn1
  PS-Simulink Converter18/LConn1 -- Spring 18/RConn2
  Spring 19/LConn1 -- X-6/RConn1 -- Revolute Joint 19/LConn1
  Y-9/RConn1 -- Spring 19/RConn1 -- End sphere 19/RConn1 -- Cable end 19/LConn1
  Spool 19/RConn1 -- Cable end 19/RConn1 -- Cable properties 19/LConn1
  Winch 19/RConn1 -- Revolute Joint 19/RConn1 -- Spool 19/LConn1
  PS-Simulink Converter19/LConn1 -- Spring 19/RConn2
  Spring 20/LConn1 -- Y+6/RConn1 -- Revolute Joint 20/LConn1
  Connection Label52/LConn1 -- X-10/LConn1
  Spool 20/RConn1 -- Cable end 20/RConn1 -- Cable properties 20/LConn1
  Winch 20/RConn1 -- Revolute Joint 20/RConn1 -- Spool 20/LConn1
  PS-Simulink Converter20/LConn1 -- Spring 20/RConn2
  Spring 21/LConn1 -- Y-7/RConn1 -- Revolute Joint 21/LConn1
  Connection Label51/LConn1 -- X+11/LConn1
  Spool 21/RConn1 -- Cable end 21/RConn1 -- Cable properties 21/LConn1
  Winch 21/RConn1 -- Revolute Joint 21/RConn1 -- Spool 21/LConn1
  PS-Simulink Converter21/LConn1 -- Spring 21/RConn2
  Spring 22/LConn1 -- X+7/RConn1 -- Revolute Joint 22/LConn1
  Y+12/RConn1 -- Spring 22/RConn1 -- End sphere 22/RConn1 -- Cable end 22/LConn1
  Spool 22/RConn1 -- Cable end 22/RConn1 -- Cable properties 22/LConn1
  Winch 22/RConn1 -- Revolute Joint 22/RConn1 -- Spool 22/LConn1
  PS-Simulink Converter22/LConn1 -- Spring 22/RConn2
  Spring 23/LConn1 -- Y-8/RConn1 -- Revolute Joint 23/LConn1
  X-9/RConn1 -- Spring 23/RConn1 -- End sphere 23/RConn1 -- Cable end 23/LConn1
  Spool 23/RConn1 -- Cable end 23/RConn1 -- Cable properties 23/LConn1
  Winch 23/RConn1 -- Revolute Joint 23/RConn1 -- Spool 23/LConn1
  PS-Simulink Converter23/LConn1 -- Spring 23/RConn2
  Spring 24/LConn1 -- X+8/RConn1 -- Revolute Joint 24/LConn1
  Connection Label48/LConn1 -- Y+10/LConn1
  Spool 24/RConn1 -- Cable end 24/RConn1 -- Cable properties 24/LConn1
  Winch 24/RConn1 -- Revolute Joint 24/RConn1 -- Spool 24/LConn1
  PS-Simulink Converter24/LConn1 -- Spring 24/RConn2
  Connection Label19/LConn1 -- X+3/LConn1
  Connection Label18/LConn1 -- Y-3/LConn1
  Connection Label17/LConn1 -- X-3/LConn1
  Connection Label16/LConn1 -- Y+3/LConn1
  X+4/RConn1 -- Revolute Joint 16/LConn1 -- Spring 16/LConn1
  Connection Label25/LConn1 -- X-4/LConn1
  Connection Label26/LConn1 -- Y-4/LConn1
  Connection Label24/LConn1 -- Y+4/LConn1
  Spring 9/RConn1 -- Y+5/RConn1 -- End sphere 9/RConn1 -- Cable end 9/LConn1
  Connection Label78/LConn1 -- Y-5/LConn1
  Connection Label33/LConn1 -- X+5/LConn1
  Revolute Joint 17/LConn1 -- X-5/RConn1 -- Spring 17/LConn1
  Connection Label34/LConn1 -- X-6/LConn1
  Connection Label69/LConn1 -- X+6/LConn1
  Connection Label37/LConn1 -- Y+6/LConn1
  Connection Label77/LConn1 -- Y-6/LConn1
  Connection Label40/LConn1 -- Y-7/LConn1
  Connection Label66/LConn1 -- Y+7/LConn1
  End sphere 5/RConn1 -- Cable end 5/LConn1 -- Spring 5/RConn1 -- X-7/RConn1
  Connection Label41/LConn1 -- X+7/LConn1
  Connection Label43/LConn1 -- X+8/LConn1
  X-8/RConn1 -- Spring 6/RConn1 -- End sphere 6/RConn1 -- Cable end 6/LConn1
  Connection Label42/LConn1 -- Y-8/LConn1
  Connection Label65/LConn1 -- Y+8/LConn1
  X+9/RConn1 -- Spring 3/RConn1 -- End sphere 3/RConn1 -- Cable end 3/LConn1
  Connection Label49/LConn1 -- X-9/LConn1
  Connection Label72/LConn1 -- Y+9/LConn1
  Connection Label53/LConn1 -- Y-9/LConn1
  Connection Label64/LConn1 -- X+10/LConn1
  End sphere 20/RConn1 -- Cable end 20/LConn1 -- X-10/RConn1 -- Spring 20/RConn1
  Y+10/RConn1 -- Spring 24/RConn1 -- End sphere 24/RConn1 -- Cable end 24/LConn1
  Connection Label68/LConn1 -- Y-10/LConn1
  End sphere 21/RConn1 -- Cable end 21/LConn1 -- X+11/RConn1 -- Spring 21/RConn1
  Connection Label75/LConn1 -- X-11/LConn1
  Spring 8/RConn1 -- Y+11/RConn1 -- End sphere 8/RConn1 -- Cable end 8/LConn1
  Y-11/RConn1 -- Spring 17/RConn1 -- End sphere 17/RConn1 -- Cable end 17/LConn1
  X+12/RConn1 -- Spring 18/RConn1 -- End sphere 18/RConn1 -- Cable end 18/LConn1
  Connection Label63/LConn1 -- X-12/LConn1
  Connection Label50/LConn1 -- Y+12/LConn1
  Connection Label67/LConn1 -- Y-12/LConn1
  Connection Label1/LConn1 -- Connection Label7/LConn1 -- Connection Label6/LConn1 -- Connection Label5/LConn1 -- Simscape Bus1/LConn1
  Rods end caps bus/RConn1 -- Simscape Bus1/RConn1
  Simscape Bus1/LConn2 -- Connection Label13/LConn1 -- Connection Label12/LConn1 -- Connection Label15/LConn1 -- Connection Label14/LConn1
  Connection Label20/LConn1 -- Connection Label23/LConn1 -- Connection Label22/LConn1 -- Connection Label21/LConn1 -- Simscape Bus1/LConn3
  Connection Label28/LConn1 -- Connection Label31/LConn1 -- Connection Label30/LConn1 -- Connection Label29/LConn1 -- Simscape Bus1/LConn4
  Connection Label32/LConn1 -- X-5/LConn1
  Connection Label84/LConn1 -- Connection Label57/LConn1 -- Connection Label61/LConn1 -- Connection Label80/LConn1 -- Simscape Bus1/LConn12
  Connection Label92/LConn1 -- Connection Label58/LConn1 -- Connection Label79/LConn1 -- Connection Label88/LConn1 -- Simscape Bus1/LConn11
  Connection Label85/LConn1 -- Connection Label55/LConn1 -- Connection Label59/LConn1 -- Connection Label81/LConn1 -- Simscape Bus1/LConn10
  Connection Label93/LConn1 -- Connection Label56/LConn1 -- Connection Label60/LConn1 -- Connection Label89/LConn1 -- Simscape Bus1/LConn9
  Connection Label90/LConn1 -- Connection Label47/LConn1 -- Connection Label46/LConn1 -- Connection Label82/LConn1 -- Simscape Bus1/LConn8
  Connection Label91/LConn1 -- Connection Label45/LConn1 -- Connection Label44/LConn1 -- Connection Label83/LConn1 -- Simscape Bus1/LConn7
  Connection Label94/LConn1 -- Connection Label39/LConn1 -- Connection Label38/LConn1 -- Connection Label86/LConn1 -- Simscape Bus1/LConn6
  Connection Label95/LConn1 -- Connection Label36/LConn1 -- Connection Label35/LConn1 -- Connection Label87/LConn1 -- Simscape Bus1/LConn5
